simulink model "Q_II_5"  (R2024b)
settings: Solver=VariableStepAuto  StartTime=0.0  StopTime=10.0  RelTol=1e-3
values from neighbouring files (symbols this model uses):
  K = (4*Jeff)/((e^2)*(Km_R))    (= 0.553333333333)    [Comm_Rob.m]
  Kd = ((4*Jeff)/(1/2) - Beff)/Km_R    (= 0.235)    [Comm_Rob.m]
  r = 1/200    (= 0.005)    [Comm_Rob.m]    (also in sf_loi_avant_RP.m; sf_retour_linearisant_boucle_interne_RP.m = 1)
  Ti = 0.8    [Comm_Rob.m]
libraries: lib_robotRP x3

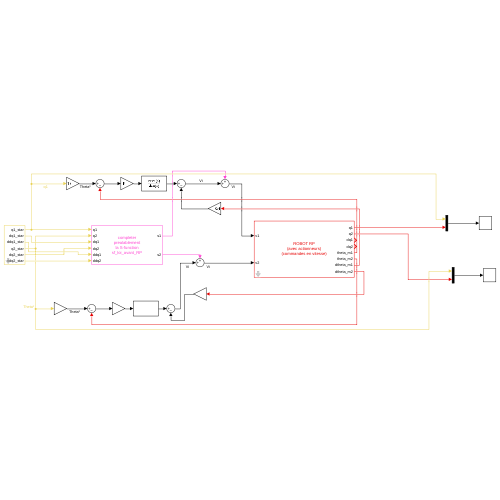
[thumbnail: Simulink's stored preview of the top-level diagram]
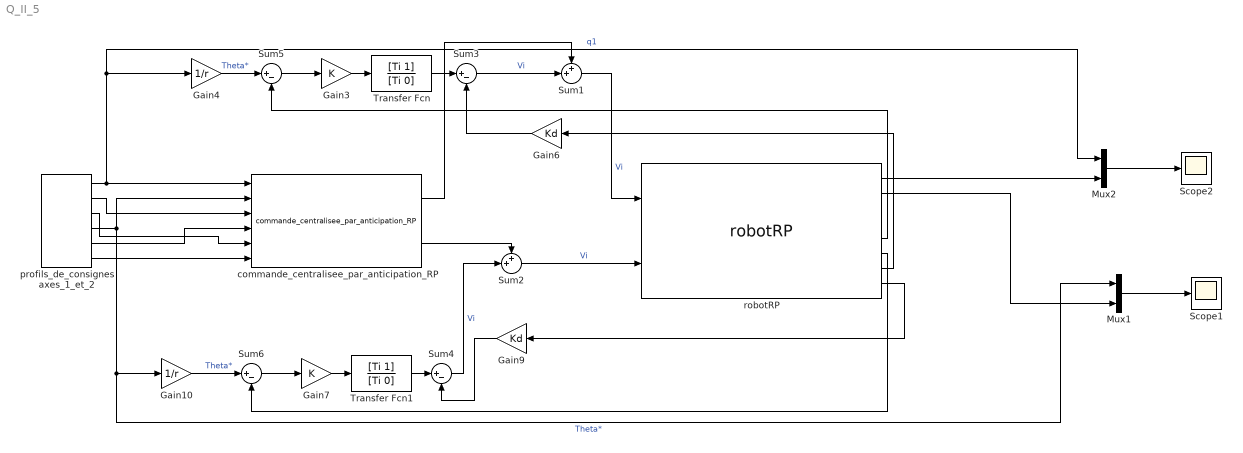
== system Q_II_5 ==
  Gain10 : Gain  Gain=1/r
  Gain3 : Gain  Gain=K
  Gain4 : Gain  Gain=1/r
  Gain6 : Gain  Gain=Kd
  Gain7 : Gain  Gain=K
  Gain9 : Gain  Gain=Kd
  Mux1 : Mux  Inputs=2
  Mux2 : Mux  Inputs=2
  Scope1 : Scope
  Scope2 : Scope
  Sum1 : Sum  Inputs=++|
  Sum2 : Sum  Inputs=++|
  Sum{3..6} (4 alike) : Sum  Inputs=|+-
  Transfer Fcn : TransferFcn  Numerator=[Ti 1]  Denominator=[Ti 0]
  Transfer Fcn1 : TransferFcn  Numerator=[Ti 1]  Denominator=[Ti 0]
  commande_centralisee_par_anticipation_RP : lib_robotRP/commande_centralisee_par_anticipation_RP  SystemSampleTime=-1  VariantActivationTime=update diagram  AllowFlexibleInterface=on  Latency=0  AutoFrameSizeCalculation=off
  profils_de_consignes axes_1_et_2 : lib_robotRP/profils_de_consignes axes_1_et_2
  robotRP : lib_robotRP/robotRP  vecteur_theta_dtheta_initial=[0 ; 0.5/r ; 0 ; 0]  m=15  gX=0  gY=-9.81  F1=0  F2=0  H1=0  H2=0  Km_sur_R=0.3  Jm=0.01  Beff=0.0125  r=r
  wires:
  Sum3/1 -> Sum1/2  "Vi"
  Sum1/1 -> robotRP/1  "Vi"
  robotRP/2 -> Mux1/2
  profils_de_consignes axes_1_et_2/4 -> Mux1/1, Gain10/1, commande_centralisee_par_anticipation_RP/2  "Theta*"
  profils_de_consignes axes_1_et_2/6 -> commande_centralisee_par_anticipation_RP/6
  Gain10/1 -> Sum6/1  "Theta*"
  Mux2/1 -> Scope2/1
  Sum6/1 -> Gain7/1
  Gain9/1 -> Sum4/2
  robotRP/8 -> Gain9/1
  profils_de_consignes axes_1_et_2/5 -> commande_centralisee_par_anticipation_RP/4
  profils_de_consignes axes_1_et_2/2 -> commande_centralisee_par_anticipation_RP/3
  Sum5/1 -> Gain3/1
  Gain3/1 -> Transfer Fcn/1
  Sum2/1 -> robotRP/2  "Vi"
  robotRP/6 -> Sum6/2
  robotRP/5 -> Sum5/2
  profils_de_consignes axes_1_et_2/3 -> commande_centralisee_par_anticipation_RP/5
  Gain7/1 -> Transfer Fcn1/1
  Gain4/1 -> Sum5/1  "Theta*"
  commande_centralisee_par_anticipation_RP/1 -> Sum1/1
  robotRP/7 -> Gain6/1
  Sum4/1 -> Sum2/2  "Vi"
  commande_centralisee_par_anticipation_RP/2 -> Sum2/1
  profils_de_consignes axes_1_et_2/1 -> Mux2/1, Gain4/1, commande_centralisee_par_anticipation_RP/1  "q1"
  Transfer Fcn/1 -> Sum3/1
  robotRP/1 -> Mux2/2
  Transfer Fcn1/1 -> Sum4/1
  Mux1/1 -> Scope1/1
  Gain6/1 -> Sum3/2
